simulink model "MySimplifiedTestingModel_20x2810x29"  (R2023a)
settings: Solver=ode1  StartTime=0.0  StopTime=inf  FixedStep=0.001  RelTol=1e-3
PostLoadFcn:
  | , if any(exist('dsrtsu_mdlpostloadfcn', 'file') ~= 0), dsrtsu_mdlpostloadfcn('Execute', bdroot); end,
InitFcn:
  | , if any(exist('rtifpga_mdlclblib', 'file') ~= 0), rtifpga_mdlclblib('Init', bdroot); end,
undefined symbols (not defined in the file or in its folder): START, STOP
libraries: rti1202serlib x11, simulink x6
(part 1 of 3)
Description:
  | Standard RTI1202 template.
  | Supported MATLAB version:  R2023a.
settings Model: Tag=RTI1202  DSRTSU_INTERNAL_RTI_VER=620  DSRTSU_INTERNAL_RTI_TYPE=rti1202  RTICANMMDATA=struct('GeneralSetupData',struct('modelroot','C:\Users\VM-User\Desktop\MigrationScripts','generalsettings',struct('filesettings',struct('destfolder',struct('Name','RTICANMM_FILES','Check',1),'buildfolder',struct('Name','.','Check',1),'AbsDestfolder',struct('Name','C:\Users\VM-User\Desktop\MigrationScripts\RTICANMM_FILES'),'AbsBuildfolder',struct('Name','C:\Users\VM-User\Desktop\MigrationScripts'))),'options',struct('addpaths',1,'rmpaths',1,'addtrcexclusion',true,'cannavigator',struct('checkmonitoring',0),'show_usrtrc',0,'use_usrtrc',0),'advanced',struct('options',ones(1,100)),'MPSetup',{{}},'RTI',struct('Type','RTI1202','Ver','7.17','Date','02-Nov-2021'),'modelname','','block','untitled'))  DSRTSU_INTERNAL_RTIFPGA=200  DSRTSU_INTERNAL_RTISTBM_VER=23.1  Creator=yd12yqyf  LastModifiedBy=ej62ixyv
settings SolverCC: AlgebraicLoopSolver=TrustRegion
settings DataIOCC: ReturnWorkspaceOutputs=off
settings OptimizationCC: BlockReduction=off  OptimizeBlockIOStorage=off  BufferReuse=off  ReuseModelBlockBuffer=off  GlobalBufferReuse=off  ExpressionFolding=off  LocalBlockOutputs=off  OptimizeDataStoreBuffers=off  BusAssignmentInplaceUpdate=off
settings DebuggingCC: UnderSpecifiedDataTypeMsg=warning  UnconnectedInputMsg=warning  UnconnectedOutputMsg=warning  UnconnectedLineMsg=warning  PregeneratedLibrarySubsystemCodeDiagnostic=none  UnderSpecifiedDimensionMsg=warning  ArithmeticOperatorsInVariantConditions=warning
settings HardwareCC: ProdBitPerPointer=32  ProdBitPerSizeT=32  ProdBitPerPtrDiffT=32  ProdLargestAtomicInteger=Integer  ProdEndianess=BigEndian  ProdWordSize=32  ProdLongLongMode=on  ProdHWDeviceType=Custom Processor->Custom  TargetIntDivRoundTo=Zero  TargetEndianess=BigEndian  TargetHWDeviceType=Custom Processor->Custom
settings ModelReferenceCC: EnableRefExpFcnMdlSchedulingChecks=on  EnableParallelModelReferenceBuilds=on  ParallelModelReferenceMATLABWorkerInit=Load Top Model
settings SFSimCC: SimUseLocalCustomCode=off  MATLABDynamicMemAlloc=off  CustomCodeUndefinedFunction=UseInterfaceOnly
settings RTWCC: Description=dSPACE DS1202 Hardware Platform  SystemTargetFile=rti1202.tlc  MakeCommand=make_rti  TemplateMakefile=rti1202.tmf  RTWUseLocalCustomCode=off  DLArmComputeVersion=19.05
settings CodeAppCC: StateflowObjectComments=on
settings STFCustomTargetCC: ParMdlRefBuildCompliant=on  ConcurrentExecutionCompliant=off  GRTInterface=off  UseToolchainInfoCompliant=off  SystemTargetFile=rti1202.tlc
settings GRTTargetCC: CompOptLevelCompliant=off  ConcurrentExecutionCompliant=off  CombineOutputUpdateFcns=off  MatFileLogging=off  CPPClassGenCompliant=off  UseToolchainInfoCompliant=off
settings ConfigComp: CovMetricSettings=dswe

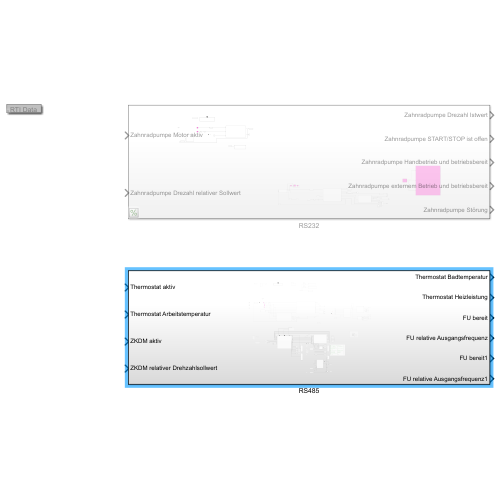
[thumbnail: Simulink's stored preview of the top-level diagram]
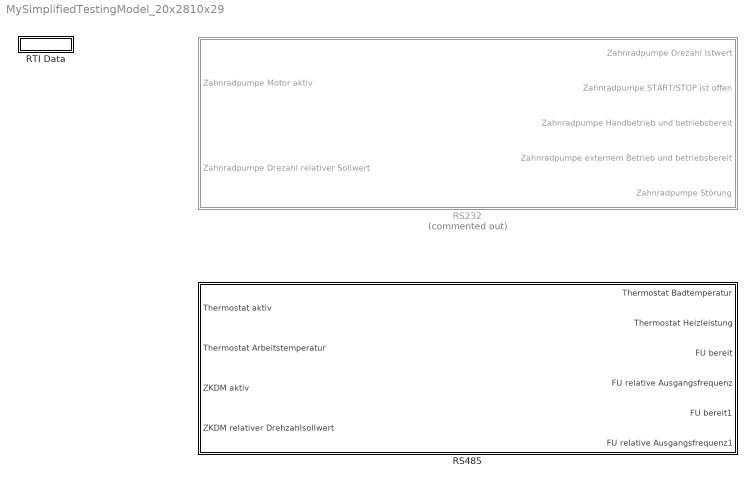
== system MySimplifiedTestingModel_20x2810x29 ==
  RS232 : Subsystem  Commented=on
  RS485 : Subsystem
  RTI Data : Subsystem  Tag=struct('RTIDataServer',struct('RTIDataServerVs','2','RTIModelDescription','struct(''main'',''MySimplifiedTestingModel_20x2810x29'',''sub'','''',''isMp'',0)'))  LoadFcn="if exist('rtidc'), try,  rtidc('DataHostBlockClbLoad', gcbh); catch, disp(['Warning: ''LoadFcn'' for RTI Data block failed: ' lasterr]); end, end,"  mask(RTI_DATA_HOST){}
      mask help:
      | RTI Data Block.
      | This block is used by RTI to store internal model-dependent data.
      | Please keep this block on the root level of the model. Deleting this block will result in data loss.
      |
      | NEVER DELETE OR COPY THIS BLOCK!
      settings: CopyFcn="if exist('rtidc'), try,  rtidc('DataHostBlockClbCopy', gcbh); catch, disp(['Warning: ''CopyFcn'' for RTI Data block failed: ' lasterr]); end, end,"  DeleteFcn="if exist('rtidc'), try,  rtidc('DataHostBlockClbDelete', gcbh); catch, disp(['Warning: ''DeleteFcn'' for RTI Data block failed: ' lasterr]); end, end,"  ModelCloseFcn="if exist('rtidc'), try,  rtidc('DataHostBlockClbModelClose', gcbh); catch, disp(['Warning: ''ModelCloseFcn'' for RTI Data block failed: ' lasterr]); end, end,"  PreSaveFcn="if exist('rtidc'), try,  rtidc('DataHostBlockClbPreSave', gcbh); catch, disp(['Warning: ''PreSaveFcn'' for RTI Data block failed: ' lasterr]); end, end,"  PostSaveFcn="if exist('rtidc'), try,  rtidc('DataHostBlockClbPostSave', gcbh); catch, disp(['Warning: ''PostSaveFcn'' for RTI Data block failed: ' lasterr]); end, end,"  NameChangeFcn="if exist('rtidc'), try,  rtidc('DataHostBlockClbNameChange', gcbh); catch, disp(['Warning: ''NameChangeFcn'' for RTI Data block failed: ' lasterr]); end, end,"
      mask Help:
      | RTI Data Block.
      | This block is used by RTI to store internal model-dependent data.
      | Please keep this block on the root level of the model. Deleting this block will result in data loss.
      | 
      | NEVER DELETE OR COPY THIS BLOCK!
      mask Display:
      | text(0.5, 0.5, 'RTI Data', 'HorizontalAlignment', 'center');
      | plot([1 0]);

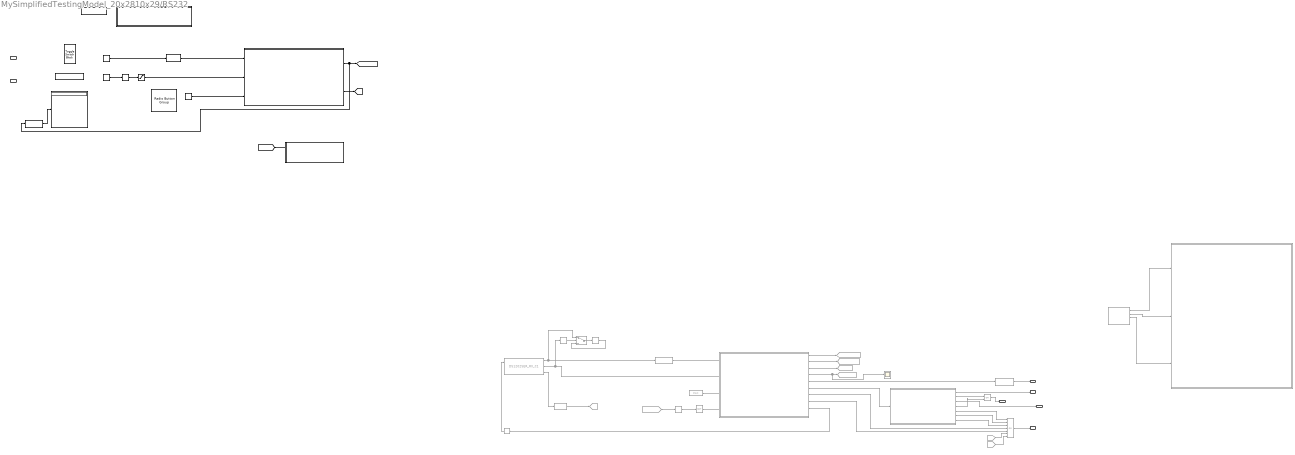
== system MySimplifiedTestingModel_20x2810x29/RS232 ==
  Zahnradpumpe Motor aktiv : Inport
  Zahnradpumpe Drezahl relativer Sollwert : Inport  Port=2
  ASCII to String : ASCIIToString  Commented=on
  ASCII to String2 : ASCIIToString
  Auswertung Statusmeldung : Subsystem  Commented=on
  Chart : Stateflow chart  TreatAsAtomicUnit=on
  Clock_in_seconds : DigitalClock  Commented=on
  Compare To Constant1 : simulink/Logic and Bit Operations/Compare To Constant  Commented=on  relop===  const=202  OutDataTypeStr=boolean
  Compare To Zero1 : simulink/Logic and Bit Operations/Compare To Zero  Commented=on  relop=>  OutDataTypeStr=boolean
  Constant : Constant  Value=0
  Create In/Out-Command Pump : Subsystem  TreatAsAtomicUnit=on
  DS1202SER_RX_C2 : rti1202serlib/DS1202SER_RX_C1  Commented=on  Reserved1=[]  Reserved2=[]  Reserved3=[]  Reserved4=[]  DSProperties=struct('RTI',struct('IOBoardType',{{'DS1202','SER'}},'SlaveProcessor','NONE','Version',uint32(1),'BlockType',struct('isSLSource',uint8(1),'isSLSink',uint8(1),'isHWSource',uint8(0),'isHWSink',uint8(1),'isSetup',uint8(0),'isInline',uint8(1),'isNonInline',uint8(0),'isInterrupt',uint8(0),'isChannelwise',uint8(1)),'UnitType','GENSER','Identifier','RECEIVE','DialogType','ML','BlockSet','NONE'))  RTIBlockInterface=struct('BlockName',struct('Token',{{'DS1202SER_RX_C'}},'BlockParam',{{'ChannelNo'}}),'InputPortsWidth',int32(1),'InputPortsActive',1,'InputPortsDataType',{{'SS_UINT32'}},'InputPortsName',{{'NumBytes'}},'OutputPortsWidth',int32([63 1 1]),'OutputPortsActive',[1 1 1],'OutputPortsDataType',{{'SS_UINT8','SS_UINT32','SS_INT32'}},'OutputPortsName',{{'RXBytes','NumRXBytes','Status'}},'BlockDisplay',{{['Serial Receive'],'center'}},'IconTransparency','on','ParameterTunableNames',{{'BytesRefNumOf'}},'InitLevel',2,'DialogFcn','guigenserreceive','MaskDescription',['To read data from the UART SW FIFO.'])  RTIBlockParameters=struct('BoardNo',{{1,'ON',[1 1]}},'ChannelNo',{{2,'ON',[1 2]}},'ChannelNumOf',{{2,'OFF',[]}},'ReceptionDataMode',{{2,'OFF',[]}},'ParamTunableMode',{{1,'OFF',[]}},'BytesRefNumOfT',{{'1','OFF',[1 inf]}},'BytesRefNumOfNT',{{'1','OFF',[1 inf]}},'BytesRefNumOfMax',{{'63','OFF',[1 inf]}},'BytesRefNumOfMode',{{0,'OFF',[]}},'BytesActNumOfMode',{{1,'OFF',[]}},'ReceptionStatusMode',{{1,'OFF',[]}},'FifoSizeDefault',{{64,'OFF',[]}},'TLCFileName',{{'rtigenserreceive','OFF',[]}})  RTISFcnParameters=struct('BoardNo','double','ChannelNo','double','ChannelNumOf','double','ReceptionDataMode','double','ParamTunableMode','double','BytesRefNumOfT','double','BytesRefNumOfNT','double','BytesRefNumOfMax','double','BytesRefNumOfMode','double','BytesActNumOfMode','double','ReceptionStatusMode','double','TLCFileName','char')  RTIBlockParaDefault=struct('BoardNo',1,'ChannelNo',1,'ChannelNumOf',2,'ReceptionDataMode',1,'ParamTunableMode',1,'BytesRefNumOfT',1,'BytesRefNumOfNT',1,'BytesRefNumOfMax',1,'BytesRefNumOfMode',0,'BytesActNumOfMode',1,'ReceptionStatusMode',1,'FifoSizeDefault',64,'TLCFileName','rtigenserreceive')
  DS1202SER_SETUP_C2 : rti1202serlib/DS1202SER_SETUP_C1  Reserved1=[]  Reserved2=[]  Reserved3=[]  Reserved4=[]  DSProperties=struct('RTI',struct('Version',uint32(2),'IOBoardType',{{'DS1202','SER'}},'SlaveProcessor','NONE','BlockType',struct('isSLSource',uint8(0),'isSLSink',uint8(0),'isHWSource',uint8(0),'isHWSink',uint8(0),'isSetup',uint8(1),'isInline',uint8(1),'isNonInline',uint8(0),'isInterrupt',uint8(0),'isChannelwise',uint8(1)),'UnitType','GENSER','Identifier','SETUP','DialogType','ML','BlockSet','NONE'))  RTIBlockInterface=struct('BlockName',struct('Token',{{'DS1202SER_SETUP_C'}},'BlockParam',{{'ChannelNo'}}),'BlockDisplay',{{['Serial Setup'],'center'}},'IconTransparency','off','ParameterTunableNames',{{}},'InitLevel',1,'DialogFcn','guigensersetup','MaskDescription',['To set the global specifications for the UART interface.'])  RTIBlockParameters=struct('ParityMode',{{1,'OFF',[1 5]}},'TransceiverMode',{{[1;1],'OFF',[]}},'QuartzFrequency',{{'160000000','OFF',[]}},'BoardNo',{{1,'ON',[1 1]}},'ChannelNo',{{2,'ON',[1 2]}},'ChannelNumOf',{{2,'OFF',[]}},'BaudRate',{{'19200','OFF',[]}},'DataBitsNumOf',{{4,'OFF',[1 4]}},'StopBitsNumOf',{{3,'OFF',[1 3]}},'ReceiveIntLevelUart',{{1,'OFF',[1 4]}},'AutoflowMode',{{0,'OFF',[]}},'FifoSize',{{'64','OFF',[]}},'ReceiveIntLevelFifo',{{0,'OFF',[]}},'FifoOverrunMode',{{1,'OFF',[]}},'FifoBlockSize',{{'0','OFF',[]}},'TermMode',{{1,'OFF',[]}},'TLCFileName',{{'rtigensersetup','OFF',[]}})  RTISFcnParameters=struct('BoardNo','double','ChannelNo','double','ChannelNumOf','double','BaudRate','double','DataBitsNumOf','double','StopBitsNumOf','double','ParityMode','double','TransceiverMode','double','ReceiveIntLevelUart','double','AutoflowMode','double','FifoSize','double','ReceiveIntLevelFifo','double','FifoBlockSize','double','TermMode','double','QuartzFrequency','double','TLCFileName','char')  RTIBlockParaDefault=struct('ParityMode',1,'TransceiverMode',[1;1],'QuartzFrequency',160000000,'BoardNo',1,'ChannelNo',1,'ChannelNumOf',2,'BaudRate',115200,'DataBitsNumOf',4,'StopBitsNumOf',1,'ReceiveIntLevelUart',4,'AutoflowMode',0,'FifoSize',64,'ReceiveIntLevelFifo',0,'FifoOverrunMode',1,'FifoBlockSize',0,'TermMode',1,'TLCFileName','rtigensersetup')
  DS1202SER_STAT_C2 : rti1202serlib/DS1202SER_STAT_C1  Commented=on  Reserved1=[]  Reserved2=[]  Reserved3=[]  Reserved4=[]  DSProperties=struct('RTI',struct('IOBoardType',{{'DS1202','SER'}},'SlaveProcessor','NONE','Version',uint32(1),'BlockType',struct('isSLSource',uint8(1),'isSLSink',uint8(0),'isHWSource',uint8(0),'isHWSink',uint8(0),'isSetup',uint8(0),'isInline',uint8(1),'isNonInline',uint8(0),'isInterrupt',uint8(0),'isChannelwise',uint8(1)),'UnitType','GENSER','Identifier','STATUS','DialogType','ML','BlockSet','NONE'))  RTIBlockInterface=struct('BlockName',struct('Token',{{'DS1202SER_STAT_C'}},'BlockParam',{{'ChannelNo'}}),'OutputPortsWidth',int32([8 8 8]),'OutputPortsActive',[1 1 1],'OutputPortsName',{{'Line','Modem','Interrupt'}},'OutputPortsDataType',{{'SS_BOOLEAN','SS_BOOLEAN','SS_BOOLEAN'}},'BlockDisplay',{{['Serial Status'],'left'}},'IconTransparency','on','ParameterTunableNames',{{}},'InitLevel',1,'DialogFcn','guigenserstatus','MaskDescription',['To read the contents of the UART status register.'])  RTIBlockParameters=struct('BoardNo',{{1,'ON',[1 1]}},'ChannelNo',{{2,'ON',[1 2]}},'ChannelNumOf',{{2,'OFF',[]}},'LineStatUartMode',{{1,'OFF',[]}},'ModemStatUartMode',{{1,'OFF',[]}},'InterruptStatUartMode',{{1,'OFF',[]}},'TLCFileName',{{'rtigenserstatus','OFF',[]}})  RTISFcnParameters=struct('BoardNo','double','ChannelNo','double','ChannelNumOf','double','LineStatUartMode','double','ModemStatUartMode','double','InterruptStatUartMode','double','TLCFileName','char')  RTIBlockParaDefault=struct('BoardNo',1,'ChannelNo',1,'ChannelNumOf',2,'LineStatUartMode',1,'ModemStatUartMode',1,'InterruptStatUartMode',1,'TLCFileName','rtigenserstatus')
  Data Type Conversion : DataTypeConversion  OutDataTypeStr=boolean  SaturateOnIntegerOverflow=off  RndMeth=Floor
  Debug RXBytes : Memory  Commented=on
  Debug Serial Status : Subsystem  Commented=on
  Display1 : Display
  Edit : EditField  LabelPosition=Hide  ShowInitialText=on  Alignment=Center
  FSM2: zyklische Datenabfrage : Stateflow chart  Commented=on  TreatAsAtomicUnit=on
  From : From  Commented=on
  From1 : From  Commented=on  GotoTag=B
  From7 : From  Commented=on  GotoTag=FSM1_Zugriff
  Goto3 : Goto  Commented=on  GotoTag=FSM2_Kommando
  Goto4 : Goto  Commented=on  GotoTag=FSM2_NumBytes
  Goto5 : Goto  Commented=on  GotoTag=TriggerTX2
  Goto6 : Goto  Commented=on  GotoTag=FSM2_Zugriff
  Logical Operator : Logic  Commented=on  Operator=OR  IconShape=distinctive  AllPortsSameDT=off  OutDataTypeStr=boolean
  Logical Operator1 : Logic  Commented=on  Operator=OR  Inputs=7  AllPortsSameDT=off  OutDataTypeStr=boolean
  Logical Operator3 : Logic  Commented=on  Operator=NOT  IconShape=distinctive  AllPortsSameDT=off  OutDataTypeStr=boolean
  Memory : Memory  Commented=on
  Memory2 : Memory  Commented=on
  RX: The FIFO is filled or not all data could be copied to the FIFO : Goto  Commented=on  GotoTag=B
  Radio Button : RadioButtonGroup  SelectedLabel=START/STOP  ButtonGroupName=Group
      settings: Values={{'START/STOP', 'STATUS'}, [0 1]}
  Round : Rounding  Operator=round
  Saturation1 : Saturate  UpperLimit=999.0  LowerLimit=0.0  RndMeth=Round
  Scope1 : Scope  Commented=on
  Sollwertvorgabe Eingang : Constant  Value=124
  Start/Stopp Eingang : Constant  Value=logical(1)
  String to Single : ScanString  Commented=on  Format="\"%d\""
  Switch2 : Switch  Commented=on  Criteria=u2 > Threshold  SaturateOnIntegerOverflow=off  InputSameDT=off
  Toggle Switch : ToggleSwitchBlock
      settings: Values={{'Off', 'On'}, [0 1]}
  Triggered Subsystem1 : Subsystem  TreatAsAtomicUnit=on
  Zahnradpumpe Drezahl Istwert : Outport
  Zahnradpumpe START/STOP ist offen : Outport  Port=2
  Zahnradpumpe Handbetrieb und betriebsbereit : Outport  Port=3
  Zahnradpumpe externem Betrieb und betriebsbereit : Outport  Port=4
  Zahnradpumpe Störung : Outport  Port=5
  wires:
  [Command] -> Triggered Subsystem1/1(Vector to send)
  Chart/2(on) -> [On]
  ASCII to String2/1 -> Display1/1
  Chart/1(Command) -> ASCII to String2/1, [Command]
  Constant/1 -> Chart/3(mode)
  Data Type Conversion/1 -> Chart/1(Pump_Start_Stop)
  FSM2: zyklische Datenabfrage/6(Statusmeldung) -> Auswertung Statusmeldung/1(Statusmeldung)
  Logical Operator/1 -> Zahnradpumpe START/STOP ist offen/1
  Auswertung Statusmeldung/2(Handbetrieb und START/STOP ist offen) -> Logical Operator/1
  Auswertung Statusmeldung/4(externem Betrieb und START/STOP ist offen) -> Logical Operator/2
  Auswertung Statusmeldung/5(Motor überhitzt) -> Logical Operator1/1
  Auswertung Statusmeldung/6(Motor nicht angeschlossen) -> Logical Operator1/2
  Auswertung Statusmeldung/7(im Modus Konfigurieren) -> Logical Operator1/3
  FSM2: zyklische Datenabfrage/7(KeineAntwort) -> Logical Operator1/4
  Logical Operator1/1 -> Zahnradpumpe Störung/1
  FSM2: zyklische Datenabfrage/9(NumBytes) -> Memory/1
  DS1202SER_RX_C2/3 -> Compare To Constant1/1
  Compare To Constant1/1 -> RX: The FIFO is filled or not all data could be copied to the FIFO/1
  From1/1 -> Logical Operator1/7
  From/1 -> Logical Operator1/6
  FSM2: zyklische Datenabfrage/8(ZykluszeitUeberschritten) -> Logical Operator1/5
  ASCII to String/1 -> FSM2: zyklische Datenabfrage/1(RXString)
  DS1202SER_RX_C2/2 -> FSM2: zyklische Datenabfrage/2(NumRXBytes), Compare To Zero1/1
  DS1202SER_RX_C2/1 -> ASCII to String/1, Switch2/1
  Memory/1 -> DS1202SER_RX_C2/1
  Debug RXBytes/1 -> Switch2/3
  Compare To Zero1/1 -> Switch2/2
  Switch2/1 -> Debug RXBytes/1
  Auswertung Statusmeldung/3(externem Betrieb und betriebsbereit) -> Zahnradpumpe externem Betrieb und betriebsbereit/1
  Auswertung Statusmeldung/1(Handbetrieb und betriebsbereit) -> Zahnradpumpe Handbetrieb und betriebsbereit/1
  DS1202SER_STAT_C2/1 -> Debug Serial Status/1(In1)
  DS1202SER_STAT_C2/2 -> Debug Serial Status/2(In2)
  DS1202SER_STAT_C2/3 -> Debug Serial Status/3(In3)
  Clock_in_seconds/1 -> FSM2: zyklische Datenabfrage/3(Clock)
  Round/1 -> Saturation1/1
  Saturation1/1 -> Chart/2(Value_numeric)
  Start/Stopp Eingang/1 -> Data Type Conversion/1
  Sollwertvorgabe Eingang/1 -> Round/1
  From7/1 -> Memory2/1
  FSM2: zyklische Datenabfrage/1(RS232_Kommando) -> Goto3/1
  FSM2: zyklische Datenabfrage/2(Kommando_NumBytes) -> Goto4/1
  FSM2: zyklische Datenabfrage/3(TriggerTX) -> Goto5/1
  FSM2: zyklische Datenabfrage/4(Zugriff) -> Scope1/1, Goto6/1
  String to Single/1 -> Zahnradpumpe Drezahl Istwert/1
  FSM2: zyklische Datenabfrage/5(Istwert) -> String to Single/1
  Memory2/1 -> Logical Operator3/1
  Logical Operator3/1 -> FSM2: zyklische Datenabfrage/4(Freigegeben)

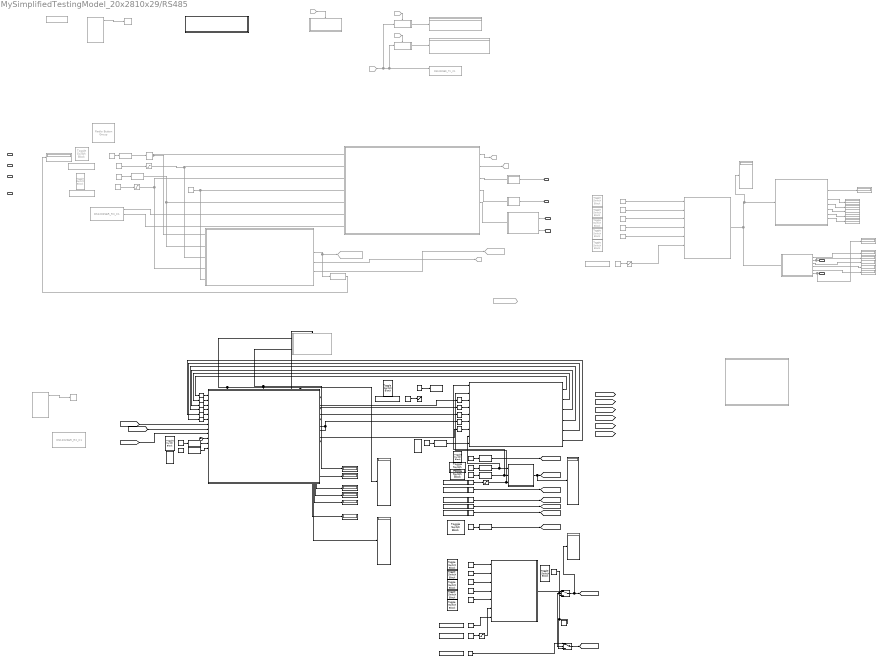
== system MySimplifiedTestingModel_20x2810x29/RS485 ==
  note: RX_Data
  note: RX_Len
  note: THRE
  note: %| Bit| Bit value = 0 | Bit value = 1 |
      | %|----|--------------------------------------|------------------------------------|
      | %| 00 | selection between the four "3-10 Preset reference [0]...[3]" |
      | %| 01 | --""-- |
      | %|----|--------------------------------------|------------------------------------|
      | %| 02 | DC brake and stop | performs ramp |
      | %|----|--------------------------------------|------------------------------------|
      | %| 03 | lets the motor coast | starts the motor if conditions are met |
      | %|----|--------------------------------------|------------------------------------|
      | %| 04 | motor speed decreases until stop | |
      | %|----|--------------------------------------|------------------------------------|
      | %| 05 | current output frequency is stored | |
      | %|----|--------------------------------------|------------------------------------|
      | %| 06 | stop using ramp time | starts the motor if conditions are met |
      | %|----|--------------------------------------|------------------------------------|
      | %| 07 | no reset | reset |
      | %|----|--------------------------------------|------------------------------------|
      | %| 08 | | output frequency "3-19 Jog [RPM]" |
      | %|----|--------------------------------------|------------------------------------|
      | %| 09 | ramp 1 active ("3-41" and "3-42") | ramp 2 active ("3-51" and "3-52") |
      | %|----|--------------------------------------|------------------------------------|
      | %| 10 | control word is ignored | control word is used |
      | %|----|--------------------------------------|------------------------------------|
      | %| 11 | relay 01 not activated | relay 01 activated |
      | %|----|--------------------------------------|------------------------------------|
      | %| 12 | relay 04 not activated | relay 04 activated |
      | %|----|--------------------------------------|------------------------------------|
      | %| 13 | parameter set selection "0-10" and "8-55" |
      | %| 14 | |
      | %|----|--------------------------------------|------------------------------------|
      | %| 15 | no reversal | reversal |
  note: expect_len_ZKDM
  note: expect_crc_kind_ZKDM
  note: expect_addr_ZKDM
  note: req_len
  note: req_bytes
  note: req_valid
  note: resp_len
  note: resp_data
  note: resp_err_ZKDM
  note: resp_ok_ZKDM
  note: grant_ZKDM
  note: tx data
  note: tx len
  note: tx trigger
  Thermostat aktiv : Inport
  Thermostat Arbeitstemperatur : Inport  Port=2  OutDataTypeStr=uint16
  ZKDM aktiv : Inport  Port=3
  ZKDM relativer Drehzahlsollwert : Inport  Port=4
  ASCII to String9 : ASCIIToString  Commented=on
  Arbeitstemperatur Thermostat : EditField  Commented=on  LabelPosition=Bottom  ShowInitialText=on  Alignment=Center
  BUS MASTER FSM : Stateflow chart  TreatAsAtomicUnit=on
      settings: PortSchema="{\"entries\":[{\"content\":{\"sides\":[{\"content\":{\"connectorIds\":[\"In4\",\"In16\",\"In18\",\"In8\",\"In14\",\"In10\",\"In1\",\"In2\",\"In3\",\"In6\",\"In11\",\"In12\",\"In5\",\"In15\",\"In17\",\"In7\",\"In13\",\"In9\"]},\"type\":\"ConnectorPlacement.EquallySpacedRectSide\",\"uuid\":\"833d115e-8081-4cb1-98c4-083d374565ad\"},{\"content\":{\"connectorIds\":[\"Out4\",\"Out6\",\"Out5\",\"Out7\",\"Out9\",\"Out10\",\"Out11\",\"Out8\"],\"side\":\"RIGHT\"},\"type\":\"ConnectorPlacement.EquallySpacedRectSide\",\"uuid\":\"f0cbf871-5cea-4f22-8059-874c69130aa3\"},{\"content\":{\"connectorIds\":[\"Out1\",\"Out2\",\"Out3\"],\"side\":\"TOP\"},\"type\":\"ConnectorPlacement.EquallySpacedRectSide\",\"uuid\":\"9def79f2-ef8f-4b80-a903-98ac734b5ab3\"}]},\"type\":\"ConnectorPlacement.EquallySpacedConnector\",\"uuid\":\"db046b19-190e-410f-b654-5051c870f3be\"}],\"packageUris\":[\"http://schema.mathworks.com/mf0/Connector/R2020b\"],\"version\":\"1.0\"}"
  Begrenzung Arbeitstemperatur : Saturate  Commented=on  UpperLimit=400  LowerLimit=70
  Begrenzung Arbeitstemperatur1 : Saturate  UpperLimit=100  LowerLimit=0  OutDataTypeStr=uint8
  Begrenzung Arbeitstemperatur2 : Saturate  Commented=on  UpperLimit=100  LowerLimit=0
  Begrenzung Arbeitstemperatur3 : Saturate  UpperLimit=100  LowerLimit=0
  Begrenzung Drehzahlsollwert : Saturate  Commented=on  UpperLimit=100  LowerLimit=0
  Bit Index 6: Transmitter holding register empty (THRE) indicator : Selector  Commented=on  InputPortWidth=8  IndexOptions=Starting index (dialog)  Indices=[6]  OutputSizes=1
  Bit Index 6: Transmitter holding register empty (THRE) indicator1 : Selector  Commented=on  InputPortWidth=8  IndexOptions=Starting index (dialog)  Indices=[6]  OutputSizes=1
  Cast To Boolean{,1..7} (8 alike) : DataTypeConversion  OutDataTypeStr=boolean  SaturateOnIntegerOverflow=off  RndMeth=Floor
  Clock : Clock
  Constant{,3,5,10,14,16..18} (8 alike) : Constant  Value=0
  Constant1 : Constant
  Constant11 : Constant  Value=34
  Constant12 : Constant  Value=8  OutDataTypeStr=uint8
  Constant13 : Constant  Value=125
  Constant15 : Constant  Value=0  OutDataTypeStr=uint8
  Constant2 : Constant  Commented=on  Value=34
  Constant4 : Constant  Value=34
  Constant6 : Constant  Value=12  OutDataTypeStr=uint8
  Constant7 : Constant  Value=31  OutDataTypeStr=uint8
  Constant8 : Constant  Value=8  OutDataTypeStr=uint8
  Constant9 : Constant  Value=6  OutDataTypeStr=uint8
  ConstantSwitch{1,3..6} (5 alike) : Constant  Commented=on
  ConstantSwitch{2,8..11} (5 alike) : Constant  Value=0
  ConstantSwitch7 : Constant
  Create 8-Bytes Command : MATLAB Function  TreatAsAtomicUnit=on
  Create FC-Protocol Command 8-Bytes : Subsystem  TreatAsAtomicUnit=on
  DS1202SER_RX_C1 : rti1202serlib/DS1202SER_RX_C1  Commented=on  Reserved1=[]  Reserved2=[]  Reserved3=[]  Reserved4=[]  DSProperties=struct('RTI',struct('IOBoardType',{{'DS1202','SER'}},'SlaveProcessor','NONE','Version',uint32(1),'BlockType',struct('isSLSource',uint8(1),'isSLSink',uint8(1),'isHWSource',uint8(0),'isHWSink',uint8(1),'isSetup',uint8(0),'isInline',uint8(1),'isNonInline',uint8(0),'isInterrupt',uint8(0),'isChannelwise',uint8(1)),'UnitType','GENSER','Identifier','RECEIVE','DialogType','ML','BlockSet','NONE'))  RTIBlockInterface=struct('BlockName',struct('Token',{{'DS1202SER_RX_C'}},'BlockParam',{{'ChannelNo'}}),'InputPortsWidth',int32(1),'InputPortsActive',1,'InputPortsDataType',{{'SS_UINT32'}},'InputPortsName',{{'NumBytes'}},'OutputPortsWidth',int32([63 1 1]),'OutputPortsActive',[1 1 1],'OutputPortsDataType',{{'SS_UINT8','SS_UINT32','SS_INT32'}},'OutputPortsName',{{'RXBytes','NumRXBytes','Status'}},'BlockDisplay',{{['Serial Receive'],'center'}},'IconTransparency','on','ParameterTunableNames',{{'BytesRefNumOf'}},'InitLevel',2,'DialogFcn','guigenserreceive','MaskDescription',['To read data from the UART SW FIFO.'])  RTIBlockParameters=struct('BoardNo',{{1,'ON',[1 1]}},'ChannelNo',{{1,'ON',[1 2]}},'ChannelNumOf',{{2,'OFF',[]}},'ReceptionDataMode',{{2,'OFF',[]}},'ParamTunableMode',{{1,'OFF',[]}},'BytesRefNumOfT',{{'1','OFF',[1 inf]}},'BytesRefNumOfNT',{{'1','OFF',[1 inf]}},'BytesRefNumOfMax',{{'63','OFF',[1 inf]}},'BytesRefNumOfMode',{{0,'OFF',[]}},'BytesActNumOfMode',{{1,'OFF',[]}},'ReceptionStatusMode',{{1,'OFF',[]}},'FifoSizeDefault',{{64,'OFF',[]}},'TLCFileName',{{'rtigenserreceive','OFF',[]}})  RTISFcnParameters=struct('BoardNo','double','ChannelNo','double','ChannelNumOf','double','ReceptionDataMode','double','ParamTunableMode','double','BytesRefNumOfT','double','BytesRefNumOfNT','double','BytesRefNumOfMax','double','BytesRefNumOfMode','double','BytesActNumOfMode','double','ReceptionStatusMode','double','TLCFileName','char')  RTIBlockParaDefault=struct('BoardNo',1,'ChannelNo',1,'ChannelNumOf',2,'ReceptionDataMode',1,'ParamTunableMode',1,'BytesRefNumOfT',1,'BytesRefNumOfNT',1,'BytesRefNumOfMax',1,'BytesRefNumOfMode',0,'BytesActNumOfMode',1,'ReceptionStatusMode',1,'FifoSizeDefault',64,'TLCFileName','rtigenserreceive')
  DS1202SER_RX_C2 : rti1202serlib/DS1202SER_RX_C1  Commented=on  Reserved1=[]  Reserved2=[]  Reserved3=[]  Reserved4=[]  DSProperties=struct('RTI',struct('IOBoardType',{{'DS1202','SER'}},'SlaveProcessor','NONE','Version',uint32(1),'BlockType',struct('isSLSource',uint8(1),'isSLSink',uint8(1),'isHWSource',uint8(0),'isHWSink',uint8(1),'isSetup',uint8(0),'isInline',uint8(1),'isNonInline',uint8(0),'isInterrupt',uint8(0),'isChannelwise',uint8(1)),'UnitType','GENSER','Identifier','RECEIVE','DialogType','ML','BlockSet','NONE'))  RTIBlockInterface=struct('BlockName',struct('Token',{{'DS1202SER_RX_C'}},'BlockParam',{{'ChannelNo'}}),'InputPortsWidth',int32(1),'InputPortsActive',1,'InputPortsDataType',{{'SS_UINT32'}},'InputPortsName',{{'NumBytes'}},'OutputPortsWidth',int32([63 1 1]),'OutputPortsActive',[1 1 1],'OutputPortsDataType',{{'SS_UINT8','SS_UINT32','SS_INT32'}},'OutputPortsName',{{'RXBytes','NumRXBytes','Status'}},'BlockDisplay',{{['Serial Receive'],'center'}},'IconTransparency','on','ParameterTunableNames',{{'BytesRefNumOf'}},'InitLevel',2,'DialogFcn','guigenserreceive','MaskDescription',['To read data from the UART SW FIFO.'])  RTIBlockParameters=struct('BoardNo',{{1,'ON',[1 1]}},'ChannelNo',{{2,'ON',[1 2]}},'ChannelNumOf',{{2,'OFF',[]}},'ReceptionDataMode',{{2,'OFF',[]}},'ParamTunableMode',{{1,'OFF',[]}},'BytesRefNumOfT',{{'1','OFF',[1 inf]}},'BytesRefNumOfNT',{{'1','OFF',[1 inf]}},'BytesRefNumOfMax',{{'63','OFF',[1 inf]}},'BytesRefNumOfMode',{{0,'OFF',[]}},'BytesActNumOfMode',{{1,'OFF',[]}},'ReceptionStatusMode',{{1,'OFF',[]}},'FifoSizeDefault',{{64,'OFF',[]}},'TLCFileName',{{'rtigenserreceive','OFF',[]}})  RTISFcnParameters=struct('BoardNo','double','ChannelNo','double','ChannelNumOf','double','ReceptionDataMode','double','ParamTunableMode','double','BytesRefNumOfT','double','BytesRefNumOfNT','double','BytesRefNumOfMax','double','BytesRefNumOfMode','double','BytesActNumOfMode','double','ReceptionStatusMode','double','TLCFileName','char')  RTIBlockParaDefault=struct('BoardNo',1,'ChannelNo',1,'ChannelNumOf',2,'ReceptionDataMode',1,'ParamTunableMode',1,'BytesRefNumOfT',1,'BytesRefNumOfNT',1,'BytesRefNumOfMax',1,'BytesRefNumOfMode',0,'BytesActNumOfMode',1,'ReceptionStatusMode',1,'FifoSizeDefault',64,'TLCFileName','rtigenserreceive')
  DS1202SER_SETUP_C1 : rti1202serlib/DS1202SER_SETUP_C1  Commented=on  Reserved1=[]  Reserved2=[]  Reserved3=[]  Reserved4=[]  DSProperties=struct('RTI',struct('Version',uint32(2),'IOBoardType',{{'DS1202','SER'}},'SlaveProcessor','NONE','BlockType',struct('isSLSource',uint8(0),'isSLSink',uint8(0),'isHWSource',uint8(0),'isHWSink',uint8(0),'isSetup',uint8(1),'isInline',uint8(1),'isNonInline',uint8(0),'isInterrupt',uint8(0),'isChannelwise',uint8(1)),'UnitType','GENSER','Identifier','SETUP','DialogType','ML','BlockSet','NONE'))  RTIBlockInterface=struct('BlockName',struct('Token',{{'DS1202SER_SETUP_C'}},'BlockParam',{{'ChannelNo'}}),'BlockDisplay',{{['Serial Setup'],'center'}},'IconTransparency','off','ParameterTunableNames',{{}},'InitLevel',1,'DialogFcn','guigensersetup','MaskDescription',['To set the global specifications for the UART interface.'])  RTIBlockParameters=struct('ParityMode',{{3,'OFF',[1 5]}},'TransceiverMode',{{[3;1],'OFF',[]}},'QuartzFrequency',{{'160000000','OFF',[]}},'BoardNo',{{1,'ON',[1 1]}},'ChannelNo',{{1,'ON',[1 2]}},'ChannelNumOf',{{2,'OFF',[]}},'BaudRate',{{'9600','OFF',[]}},'DataBitsNumOf',{{3,'OFF',[1 4]}},'StopBitsNumOf',{{1,'OFF',[1 3]}},'ReceiveIntLevelUart',{{1,'OFF',[1 4]}},'AutoflowMode',{{0,'OFF',[]}},'FifoSize',{{'64','OFF',[]}},'ReceiveIntLevelFifo',{{0,'OFF',[]}},'FifoOverrunMode',{{1,'OFF',[]}},'FifoBlockSize',{{'0','OFF',[]}},'TermMode',{{1,'OFF',[]}},'TLCFileName',{{'rtigensersetup','OFF',[]}})  RTISFcnParameters=struct('BoardNo','double','ChannelNo','double','ChannelNumOf','double','BaudRate','double','DataBitsNumOf','double','StopBitsNumOf','double','ParityMode','double','TransceiverMode','double','ReceiveIntLevelUart','double','AutoflowMode','double','FifoSize','double','ReceiveIntLevelFifo','double','FifoBlockSize','double','TermMode','double','QuartzFrequency','double','TLCFileName','char')  RTIBlockParaDefault=struct('ParityMode',1,'TransceiverMode',[1;1],'QuartzFrequency',160000000,'BoardNo',1,'ChannelNo',1,'ChannelNumOf',2,'BaudRate',115200,'DataBitsNumOf',4,'StopBitsNumOf',1,'ReceiveIntLevelUart',4,'AutoflowMode',0,'FifoSize',64,'ReceiveIntLevelFifo',0,'FifoOverrunMode',1,'FifoBlockSize',0,'TermMode',1,'TLCFileName','rtigensersetup')
  DS1202SER_STAT_C1 : rti1202serlib/DS1202SER_STAT_C1  Commented=on  Reserved1=[]  Reserved2=[]  Reserved3=[]  Reserved4=[]  DSProperties=struct('RTI',struct('IOBoardType',{{'DS1202','SER'}},'SlaveProcessor','NONE','Version',uint32(1),'BlockType',struct('isSLSource',uint8(1),'isSLSink',uint8(0),'isHWSource',uint8(0),'isHWSink',uint8(0),'isSetup',uint8(0),'isInline',uint8(1),'isNonInline',uint8(0),'isInterrupt',uint8(0),'isChannelwise',uint8(1)),'UnitType','GENSER','Identifier','STATUS','DialogType','ML','BlockSet','NONE'))  RTIBlockInterface=struct('BlockName',struct('Token',{{'DS1202SER_STAT_C'}},'BlockParam',{{'ChannelNo'}}),'OutputPortsWidth',int32([8 8 8]),'OutputPortsActive',[1 1 1],'OutputPortsName',{{'Line','Modem','Interrupt'}},'OutputPortsDataType',{{'SS_BOOLEAN','SS_BOOLEAN','SS_BOOLEAN'}},'BlockDisplay',{{['Serial Status'],'left'}},'IconTransparency','on','ParameterTunableNames',{{}},'InitLevel',1,'DialogFcn','guigenserstatus','MaskDescription',['To read the contents of the UART status register.'])  RTIBlockParameters=struct('BoardNo',{{1,'ON',[1 1]}},'ChannelNo',{{1,'ON',[1 2]}},'ChannelNumOf',{{2,'OFF',[]}},'LineStatUartMode',{{1,'OFF',[]}},'ModemStatUartMode',{{1,'OFF',[]}},'InterruptStatUartMode',{{1,'OFF',[]}},'TLCFileName',{{'rtigenserstatus','OFF',[]}})  RTISFcnParameters=struct('BoardNo','double','ChannelNo','double','ChannelNumOf','double','LineStatUartMode','double','ModemStatUartMode','double','InterruptStatUartMode','double','TLCFileName','char')  RTIBlockParaDefault=struct('BoardNo',1,'ChannelNo',1,'ChannelNumOf',2,'LineStatUartMode',1,'ModemStatUartMode',1,'InterruptStatUartMode',1,'TLCFileName','rtigenserstatus')
  DS1202SER_STAT_C2 : rti1202serlib/DS1202SER_STAT_C1  Commented=on  Reserved1=[]  Reserved2=[]  Reserved3=[]  Reserved4=[]  DSProperties=struct('RTI',struct('IOBoardType',{{'DS1202','SER'}},'SlaveProcessor','NONE','Version',uint32(1),'BlockType',struct('isSLSource',uint8(1),'isSLSink',uint8(0),'isHWSource',uint8(0),'isHWSink',uint8(0),'isSetup',uint8(0),'isInline',uint8(1),'isNonInline',uint8(0),'isInterrupt',uint8(0),'isChannelwise',uint8(1)),'UnitType','GENSER','Identifier','STATUS','DialogType','ML','BlockSet','NONE'))  RTIBlockInterface=struct('BlockName',struct('Token',{{'DS1202SER_STAT_C'}},'BlockParam',{{'ChannelNo'}}),'OutputPortsWidth',int32([8 8 8]),'OutputPortsActive',[1 1 1],'OutputPortsName',{{'Line','Modem','Interrupt'}},'OutputPortsDataType',{{'SS_BOOLEAN','SS_BOOLEAN','SS_BOOLEAN'}},'BlockDisplay',{{['Serial Status'],'left'}},'IconTransparency','on','ParameterTunableNames',{{}},'InitLevel',1,'DialogFcn','guigenserstatus','MaskDescription',['To read the contents of the UART status register.'])  RTIBlockParameters=struct('BoardNo',{{1,'ON',[1 1]}},'ChannelNo',{{2,'ON',[1 2]}},'ChannelNumOf',{{2,'OFF',[]}},'LineStatUartMode',{{1,'OFF',[]}},'ModemStatUartMode',{{1,'OFF',[]}},'InterruptStatUartMode',{{1,'OFF',[]}},'TLCFileName',{{'rtigenserstatus','OFF',[]}})  RTISFcnParameters=struct('BoardNo','double','ChannelNo','double','ChannelNumOf','double','LineStatUartMode','double','ModemStatUartMode','double','InterruptStatUartMode','double','TLCFileName','char')  RTIBlockParaDefault=struct('BoardNo',1,'ChannelNo',1,'ChannelNumOf',2,'LineStatUartMode',1,'ModemStatUartMode',1,'InterruptStatUartMode',1,'TLCFileName','rtigenserstatus')
  DS1202SER_TX_C1 : rti1202serlib/DS1202SER_TX_C1  Commented=on  Reserved1=[]  Reserved2=[]  Reserved3=[]  Reserved4=[]  DSProperties=struct('RTI',struct('IOBoardType',{{'DS1202','SER'}},'SlaveProcessor','NONE','Version',uint32(1),'BlockType',struct('isSLSource',uint8(1),'isSLSink',uint8(1),'isHWSource',uint8(1),'isHWSink',uint8(0),'isSetup',uint8(0),'isInline',uint8(1),'isNonInline',uint8(0),'isInterrupt',uint8(0),'isChannelwise',uint8(1)),'UnitType','GENSER','Identifier','TRANSMIT','DialogType','ML','BlockSet','NONE'))  RTIBlockInterface=struct('BlockName',struct('Token',{{'DS1202SER_TX_C'}},'BlockParam',{{'ChannelNo'}}),'InputPortsWidth',int32([63 1]),'InputPortsActive',[1 1],'InputPortsDataType',{{'SS_UINT8','SS_UINT32'}},'InputPortsName',{{'TXBytes','NumBytes'}},'OutputPortsWidth',int32([1 1]),'OutputPortsActive',[0 1],'OutputPortsDataType',{{'SS_UINT32','SS_INT32'}},'OutputPortsName',{{'NumTXBytes','Status'}},'BlockDisplay',{{['Serial Transmit'],'center'}},'IconTransparency','on','ParameterTunableNames',{{'BytesRefNumOf'}},'InitLevel',2,'DialogFcn','guigensertransmit','MaskDescription',['To write data to the UART SW FIFO.'])  RTIBlockParameters=struct('BoardNo',{{1,'ON',[1 1]}},'ChannelNo',{{1,'ON',[1 2]}},'ChannelNumOf',{{2,'OFF',[]}},'TransmitFifoOverrunMode',{{1,'OFF',[]}},'ParamTunableMode',{{1,'OFF',[]}},'BytesRefNumOfT',{{'1','OFF',[1 inf]}},'BytesRefNumOfNT',{{'1','OFF',[1 inf]}},'BytesRefNumOfMax',{{'63','OFF',[1 inf]}},'BytesRefNumOfMode',{{0,'OFF',[]}},'BytesActNumOfMode',{{0,'OFF',[]}},'TransmissionStatusMode',{{1,'OFF',[]}},'FifoSizeDefault',{{64,'OFF',[]}},'TLCFileName',{{'rtigensertransmit','OFF',[]}})  RTISFcnParameters=struct('BoardNo','double','ChannelNo','double','ChannelNumOf','double','TransmitFifoOverrunMode','double','ParamTunableMode','double','BytesRefNumOfT','double','BytesRefNumOfNT','double','BytesRefNumOfMax','double','BytesRefNumOfMode','double','BytesActNumOfMode','double','TransmissionStatusMode','double','TLCFileName','char')  RTIBlockParaDefault=struct('BoardNo',1,'ChannelNo',1,'ChannelNumOf',2,'TransmitFifoOverrunMode',1,'ParamTunableMode',1,'BytesRefNumOfT',1,'BytesRefNumOfNT',1,'BytesRefNumOfMax',1,'BytesRefNumOfMode',0,'BytesActNumOfMode',1,'TransmissionStatusMode',1,'FifoSizeDefault',64,'TLCFileName','rtigensertransmit')
  Data Type Conversion : DataTypeConversion  Commented=on  OutDataTypeStr=boolean  SaturateOnIntegerOverflow=off  RndMeth=Floor
  Data Type Conversion2 : DataTypeConversion  Commented=on  OutDataTypeStr=boolean  SaturateOnIntegerOverflow=off  RndMeth=Floor
  Display{,1..15} (16 alike) : Display  Commented=on
      Display15 settings: Decimation=8
  Display{16..25} (10 alike) : Display
      Display19 settings: Decimation=16
      Display21 settings: Decimation=16
      Display22 settings: Decimation=16
      Display25 settings: Decimation=8
  Edit{,3..10} (9 alike) : EditField  LabelPosition=Hide  ShowInitialText=on  Alignment=Center
  Edit1 : EditField  Commented=on  LabelPosition=Bottom  ShowInitialText=on  Alignment=Center
  Edit2 : EditField  Commented=on  LabelPosition=Hide  ShowInitialText=on  Alignment=Center
  From : From  Commented=on  GotoTag=Command
  From1 : From  Commented=on  GotoTag=Thermostat
  From2 : From  Commented=on  GotoTag=ZKDM
  From36 : From  Commented=on  GotoTag=FSM3_RX_NumBytes
  From41 : From  Commented=on  GotoTag=ZKDM
  Goto : Goto  Commented=on  GotoTag=Command
  Goto21 : Goto  Commented=on  GotoTag=Thermostat
  Goto22 : Goto  Commented=on  GotoTag=ZKDM
  Goto23 : Goto  Commented=on  GotoTag=RS485_Kommando
  Goto24 : Goto  Commented=on  GotoTag=NumBytes
  IC : InitialCondition  Commented=on  Value=false
  Konfiguration für kommunikation ZKDM : Subsystem  Commented=on  TreatAsAtomicUnit=on
  MATLAB Function : MATLAB Function  Commented=on  TreatAsAtomicUnit=on
  MATLAB Function1 : MATLAB Function  Commented=on  TreatAsAtomicUnit=on
  MATLAB Function2 : MATLAB Function  Commented=on  TreatAsAtomicUnit=on
  MATLAB Function3 : MATLAB Function  Commented=on  TreatAsAtomicUnit=on
  MATLAB Function4 : MATLAB Function  TreatAsAtomicUnit=on
  Memory{,1..10} (11 alike) : Memory
  Mode selection : Constant  Commented=on
  Need to test the Status commands : Stateflow chart  Commented=on  TreatAsAtomicUnit=on
      settings: PortSchema="{\"entries\":[{\"content\":{\"sides\":[{\"content\":{\"connectorIds\":[\"In1\",\"In2\",\"In3\",\"In4\",\"In5\",\"In7\",\"In6\"]},\"type\":\"ConnectorPlacement.EquallySpacedRectSide\",\"uuid\":\"2bc79b64-b3a7-4950-ab47-fe1242bf0e7b\"},{\"content\":{\"connectorIds\":[\"Out1\",\"Out2\",\"Out3\",\"Out4\",\"Out5\",\"Out6\",\"Out7\"],\"side\":\"RIGHT\"},\"type\":\"ConnectorPlacement.EquallySpacedRectSide\",\"uuid\":\"7c2eb613-d548-49c2-a5a7-d00d82440fa6\"},{\"content\":{\"side\":\"TOP\"},\"type\":\"ConnectorPlacement.EquallySpacedRectSide\",\"uuid\":\"3decab41-5b6e-4ba6-8d62-f2be0ed54649\"}]},\"type\":\"ConnectorPlacement.EquallySpacedConnector\",\"uuid\":\"706bbc92-af32-40e6-b805-9cedd6f5acf9\"}],\"packageUris\":[\"http://schema.mathworks.com/mf0/Connector/R2020b\"],\"version\":\"1.0\"}"
  Radio Button : RadioButtonGroup  Commented=on  SelectedLabel=ZKDM  ButtonGroupName=Group
      settings: Values={{'Thermo', 'ZKDM', 'Status Thermo', 'Status ZKDM'}, [0 1 2 3]}
  Saturation : Saturate  UpperLimit=100  LowerLimit=0  OutDataTypeStr=uint8
  Subsystem : Subsystem  Commented=on
  Subsystem1 : Subsystem  Commented=on
  Subsystem2 : Subsystem  Commented=on
  Switch : Switch  Criteria=u2 > Threshold  SaturateOnIntegerOverflow=off  InputSameDT=off
  Switch1 : Switch  Criteria=u2 > Threshold  SaturateOnIntegerOverflow=off  InputSameDT=off
  THERMO FSM : Stateflow chart  Commented=on  TreatAsAtomicUnit=on
  Testing only Sending ON/OFF and Value commands : Stateflow chart  Commented=on  TreatAsAtomicUnit=on
  Thermostat_Arbeitstemperatur : Constant  Commented=on  Value=123
  Thermostat_StartStopp : Constant  Commented=on  Value=0  OutMin=0  OutMax=1
  Toggle Switch{,1,3..7} (7 alike) : ToggleSwitchBlock  Commented=on
      settings: Values={{'Off', 'On'}, [0 1]}
  Toggle Switch{2,8..20} (14 alike) : ToggleSwitchBlock
      settings: Values={{'Off', 'On'}, [0 1]}
  Triggered Subsystem : Subsystem  Commented=on  TreatAsAtomicUnit=on
  Triggered Subsystem1 : Subsystem  Commented=on  TreatAsAtomicUnit=on
  ZKDM FSM : Stateflow chart  TreatAsAtomicUnit=on
  ZKDM_Drehzahlsollwert : Constant  Commented=on  Value=120
  ZKDM_StartStopp : Constant  Commented=on  Value=0  OutMin=0  OutMax=1
  " Thermostat Badtemperatur" : Outport
  Thermostat Heizleistung : Outport  Port=2
  FU bereit : Outport  Port=3
  FU relative Ausgangsfrequenz : Outport  Port=4
  FU bereit1 : Outport  Port=5
  FU relative Ausgangsfrequenz1 : Outport  Port=6
  wires:
  Thermostat_StartStopp/1 -> Data Type Conversion/1
  Thermostat_Arbeitstemperatur/1 -> Begrenzung Arbeitstemperatur/1
  ZKDM_Drehzahlsollwert/1 -> Begrenzung Drehzahlsollwert/1
  ZKDM_StartStopp/1 -> Data Type Conversion2/1
  DS1202SER_STAT_C1/1 -> Bit Index 6: Transmitter holding register empty (THRE) indicator/1
  Data Type Conversion/1 -> IC/1
  IC/1 -> Need to test the Status commands/1(Start_Stop), Testing only Sending ON/OFF and Value commands/1(Start_Stop)
  Mode selection/1 -> Testing only Sending ON/OFF and Value commands/5(select), Need to test the Status commands/4(select)
  DS1202SER_RX_C2/1 -> Need to test the Status commands/7(RXVector)
  Need to test the Status commands/5(ZKDMZustand) -> Subsystem1/1(Antworttelegramm)
  Subsystem1/2(FU bereit) -> FU bereit/1
  Subsystem1/6(relative Ausgangsfrequenz) -> FU relative Ausgangsfrequenz/1
  Need to test the Status commands/3(ThermostatBadtemperatur) -> MATLAB Function/1(u)
  MATLAB Function/1(y) -> " Thermostat Badtemperatur"/1
  Need to test the Status commands/4(ThermostatHeizleistung) -> MATLAB Function1/1(u)
  MATLAB Function1/1(y) -> Thermostat Heizleistung/1
  Begrenzung Arbeitstemperatur/1 -> Testing only Sending ON/OFF and Value commands/3(Temperature_value), Need to test the Status commands/2(Temperature_value)
  Data Type Conversion2/1 -> Testing only Sending ON/OFF and Value commands/2(Start_Stop2), Need to test the Status commands/5(Start_Stop2)
  Begrenzung Drehzahlsollwert/1 -> Need to test the Status commands/3(ZKDM_value), Testing only Sending ON/OFF and Value commands/4(ZKDM_value)
  DS1202SER_RX_C2/2 -> Need to test the Status commands/6(RXBytes)
  From41/1 -> Konfiguration für kommunikation ZKDM/Trigger
  Need to test the Status commands/1(RS485_Kommando) -> Goto23/1
  Need to test the Status commands/2(NumBytes) -> Goto24/1
  Testing only Sending ON/OFF and Value commands/3(RS485_Kommando) -> Goto/1, ASCII to String9/1
  ASCII to String9/1 -> Display9/1
  Testing only Sending ON/OFF and Value commands/5(accthermo) -> Goto21/1
  Testing only Sending ON/OFF and Value commands/4(acc2) -> Goto22/1
  From1/1 -> Triggered Subsystem/Trigger
  Triggered Subsystem/1(useroutput) -> Display/1
  From2/1 -> Triggered Subsystem1/Trigger
  Triggered Subsystem1/1(y) -> Display1/1
  From/1 -> DS1202SER_TX_C1/1, Triggered Subsystem1/1(u), Triggered Subsystem/1(In1)
  Constant1/1 -> Begrenzung Arbeitstemperatur1/1
  DS1202SER_STAT_C2/1 -> Bit Index 6: Transmitter holding register empty (THRE) indicator1/1
  Clock/1 -> BUS MASTER FSM/6(now)
  BUS MASTER FSM/4(grant_ZKDM) -> Memory/1, Display16/1
  BUS MASTER FSM/6(resp_ok_ZKDM) -> Memory1/1, Display17/1
  BUS MASTER FSM/5(resp_err_ZKDM) -> Memory2/1, Display18/1
  BUS MASTER FSM/7(resp_data) -> Display19/1, Memory3/1
  BUS MASTER FSM/9(resp_len) -> Memory4/1, Display20/1
  BUS MASTER FSM/1(TX_Data) -> Subsystem/1(TXBytes), Display22/1
  BUS MASTER FSM/2(TX_Len) -> Subsystem/2(NumBytes), Display23/1
  BUS MASTER FSM/3(TX_Trigger) -> Subsystem/Trigger, Display24/1
  ZKDM FSM/1(req_valid) -> Memory5/1
  ZKDM FSM/2(req_bytes) -> Memory6/1
  ZKDM FSM/3(req_len) -> Memory7/1
  ZKDM FSM/4(expect_addr_ZKDM) -> Memory8/1
  ZKDM FSM/6(expect_len_ZKDM) -> Memory9/1
  ZKDM FSM/5(expect_crc_kind_ZKDM) -> Memory10/1
  MATLAB Function3/1(u) -> Subsystem2/1(Antworttelegramm), Display15/1, MATLAB Function2/1(u)
  Begrenzung Arbeitstemperatur2/1 -> MATLAB Function3/6(freq_rel_percent)
  Constant2/1 -> Begrenzung Arbeitstemperatur2/1
  ConstantSwitch1/1 -> MATLAB Function3/1(fu_ctrl_ready)
  ConstantSwitch3/1 -> MATLAB Function3/2(fu_ready)
  ConstantSwitch4/1 -> MATLAB Function3/3(fault_trip)
  ConstantSwitch5/1 -> MATLAB Function3/4(fault_no_trip)
  ConstantSwitch6/1 -> MATLAB Function3/5(bus_control_active)
  MATLAB Function2/3(freq_rel_percent) -> Display2/1
  MATLAB Function2/5(fu_ctrl_ready) -> Display3/1
  MATLAB Function2/6(fu_ready) -> Display4/1
  MATLAB Function2/7(fault_trip) -> Display5/1
  MATLAB Function2/8(fault_no_trip) -> Display6/1
  MATLAB Function2/9(bus_control_active) -> Display7/1
  Subsystem2/5(Bussteuerung aktive) -> Display14/1
  Subsystem2/2(FU bereit) -> Display11/1, FU bereit1/1
  Subsystem2/1(Steuerung FU bereit) -> Display10/1
  Subsystem2/6(relative Ausgangsfrequenz) -> Display8/1, FU relative Ausgangsfrequenz1/1
  Subsystem2/3(Fehler mit Abschaltung) -> Display12/1
  Subsystem2/4(Fehler ohne Abschaltung) -> Display13/1
  Cast To Boolean/1 -> ZKDM FSM/8(invalid_flag), Create 8-Bytes Command/1(invalid_flag)
  Cast To Boolean1/1 -> ZKDM FSM/1(active), Create 8-Bytes Command/2(active)
  Saturation/1 -> ZKDM FSM/2(setpoint), Create 8-Bytes Command/3(setpoint)
  Constant/1 -> Cast To Boolean/1
  Constant3/1 -> Cast To Boolean1/1
  Constant4/1 -> Saturation/1
  Constant5/1 -> Cast To Boolean2/1
  Constant6/1 -> [expect_addr_ZKDM]
  Constant7/1 -> [expect_crc_kind_ZKDM]
  Constant8/1 -> [expect_len_ZKDM]
  Constant9/1 -> [req_len]
  Cast To Boolean2/1 -> [req_valid]
  Create 8-Bytes Command/1(command) -> Display21/1, [req_bytes]
  Cast To Boolean3/1 -> [THRE]
  Constant10/1 -> Cast To Boolean3/1
  Begrenzung Arbeitstemperatur3/1 -> MATLAB Function4/6(freq_rel_percent)
  ConstantSwitch10/1 -> MATLAB Function4/4(fault_no_trip)
  ConstantSwitch8/1 -> MATLAB Function4/2(fu_ready)
  ConstantSwitch11/1 -> MATLAB Function4/5(bus_control_active)
  Constant11/1 -> Begrenzung Arbeitstemperatur3/1
  ConstantSwitch7/1 -> MATLAB Function4/1(fu_ctrl_ready)
  MATLAB Function4/1(u) -> Switch/1
  ConstantSwitch9/1 -> MATLAB Function4/3(fault_trip)
  Constant12/1 -> Switch1/1
  [THRE] -> BUS MASTER FSM/1(THRE)
  [RX_Data] -> BUS MASTER FSM/2(RX_Data)
  [RX_Len] -> BUS MASTER FSM/3(RX_Len)
  Constant13/1 -> MATLAB Function4/7(addr)
  Switch/1 -> Display25/1, [RX_Data]
  Constant14/1 -> Switch1/2, Switch/2
  Constant15/1 -> Switch1/3, Switch/3
  Switch1/1 -> [RX_Len]
  ConstantSwitch2/1 -> Cast To Boolean4/1
  Memory1/1 -> ZKDM FSM/4(resp_ok)
  Memory/1 -> ZKDM FSM/3(grant)
  Memory2/1 -> ZKDM FSM/5(resp_err)
  Memory3/1 -> ZKDM FSM/6(resp_data)
  Memory4/1 -> ZKDM FSM/7(resp_len)
  Memory5/1 -> BUS MASTER FSM/4(req_valid_ZKDM)
  Memory6/1 -> BUS MASTER FSM/16(req_bytes_ZKDM)
  Memory7/1 -> BUS MASTER FSM/18(req_len_ZKDM)
  Memory8/1 -> BUS MASTER FSM/8(expect_addr_ZKDM)
  Memory9/1 -> BUS MASTER FSM/14(expect_len_ZKDM)
  Memory10/1 -> BUS MASTER FSM/10(expect_crc_kind_ZKDM)
  Constant16/1 -> Cast To Boolean5/1
  Cast To Boolean5/1 -> ZKDM FSM/9(tx_trigger)
  Cast To Boolean6/1 -> BUS MASTER FSM/11(tx_switch)
  Constant17/1 -> Cast To Boolean6/1
  Cast To Boolean7/1 -> BUS MASTER FSM/12(rx_switch)

== system MySimplifiedTestingModel_20x2810x29/RTI Data ==
  RTI Data Store : Subsystem  Tag="struct('private',struct('version',struct('dsVer',uint32(2)),'access',struct('modified',['08-Dec-2025 11:40:10'],'type','Model','isPerm',1)),'public',struct('main',struct('data',[]),'sub',struct('name',{{'MySimplifiedTestingModel_20x2810x29'}},'data',{{struct('TH',struct('thTaskInfo',struct('taskType',{'TIMER','HWINT','TMRINT','SWINT','GLINT'},'tasksNumOf',{1,0,0,0,0},'srcIds',{{'TIMERA'},{},{},{},{}},'taskNames',{{['Timer Task 1']},{},{},{},{}})),'th_tc',struct('dataType','TASK','taskGroupId','','taskGroupList',{{}},'taskSchedulingPolicy','FCFS','taskType','TIMER','blkh',-1,'srcId','TIMERA','srcSgnName',['Timer A interrupt'],'srcCpuName','','taskName',['Timer Task 1  [0.001] s'],'taskNameDisplayExt','','smplTime',0.001,'smplTimeOffs',0,'hasFixedPriority',0,'priority',1,'hasFixedOvc',0,'ovcType',1,'ovcMax',1),'tc_th',struct('dataType','TASK','taskGroupId','','taskGroupList',{{}},'taskSchedulingPolicy','FCFS','taskType','TIMER','blkh',-1,'srcId','TIMERA','srcSgnName',['Timer A interrupt'],'srcCpuName','','taskName',['Timer Task 1  [0.001] s'],'taskNameDisplayExt','','smplTime',0.001,'smplTimeOffs',0,'hasFixedPriority',0,'priority',1,'hasFixedOvc',0,'ovcType',1,'ovcMax',1))}})))"  mask(RTI_DATA_STORE){}
      mask help:
      | RTI Data Store Block. This block is used by RTI to store internal model dependent data. Deleting this block will result in data loss.
      |
      | NEVER DELETE, COPY, OR MODIFY THIS BLOCK!
      mask Help:
      | RTI Data Store Block. This block is used by RTI to store internal model dependent data. Deleting this block will result in data loss.
      | 
      | NEVER DELETE, COPY, OR MODIFY THIS BLOCK!
      mask Display: text(0.5, 0.5, ' ', 'HorizontalAlignment', 'center');

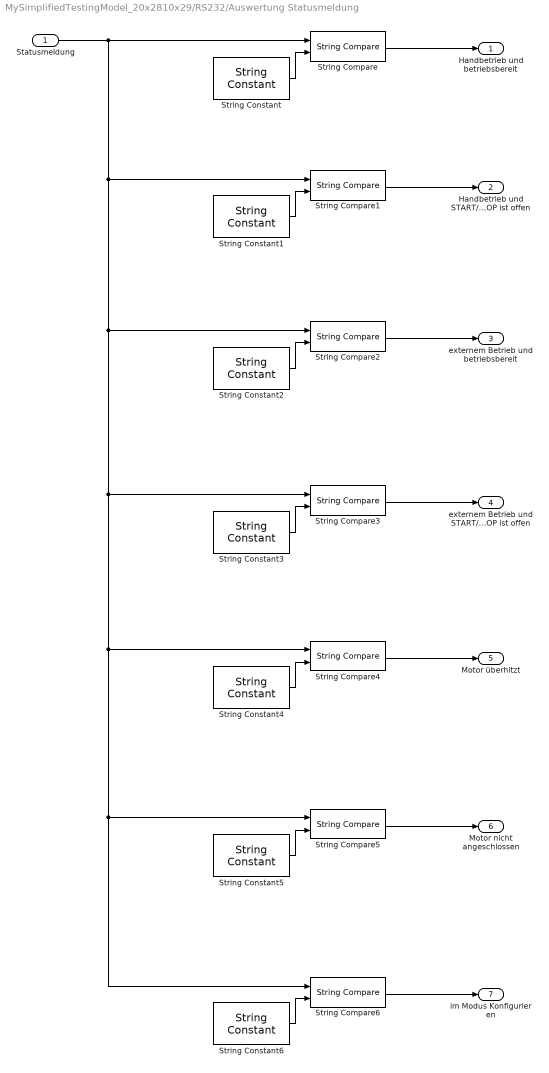
== system MySimplifiedTestingModel_20x2810x29/RS232/Auswertung Statusmeldung ==
  Statusmeldung : Inport
  String Compare{,1..6} (7 alike) : StringCompare
  String Constant : StringConstant  String="\"0\""
  String Constant1 : StringConstant  String="\"1\""
  String Constant2 : StringConstant  String="\"2\""
  String Constant3 : StringConstant  String="\"3\""
  String Constant4 : StringConstant  String="\"6\""
  String Constant5 : StringConstant  String="\"7\""
  String Constant6 : StringConstant  String="\"8\""
  Handbetrieb und betriebsbereit : Outport
  Handbetrieb und START/STOP ist offen : Outport  Port=2
  externem Betrieb und betriebsbereit : Outport  Port=3
  externem Betrieb und START/STOP ist offen : Outport  Port=4
  Motor überhitzt : Outport  Port=5
  Motor nicht angeschlossen : Outport  Port=6
  im Modus Konfigurieren : Outport  Port=7
  wires:
  String Constant/1 -> String Compare/2
  String Compare/1 -> Handbetrieb und betriebsbereit/1
  String Constant1/1 -> String Compare1/2
  String Compare1/1 -> Handbetrieb und START/STOP ist offen/1
  String Constant2/1 -> String Compare2/2
  String Compare2/1 -> externem Betrieb und betriebsbereit/1
  String Constant3/1 -> String Compare3/2
  String Compare3/1 -> externem Betrieb und START/STOP ist offen/1
  String Constant4/1 -> String Compare4/2
  String Compare4/1 -> Motor überhitzt/1
  String Constant5/1 -> String Compare5/2
  String Compare5/1 -> Motor nicht angeschlossen/1
  String Constant6/1 -> String Compare6/2
  String Compare6/1 -> im Modus Konfigurieren/1
  Statusmeldung/1 -> String Compare6/1, String Compare5/1, String Compare4/1, String Compare3/1, String Compare2/1, String Compare1/1, String Compare/1
